simulink model "LQR"  (R2024b)
settings: Solver=VariableStepAuto  StartTime=0.0  StopTime=20  RelTol=1e-3
settings Model: Creator=12625  LastModifiedBy=12625

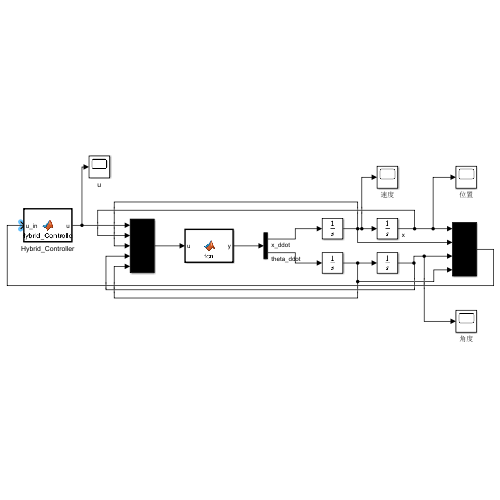
[thumbnail: Simulink's stored preview of the top-level diagram]
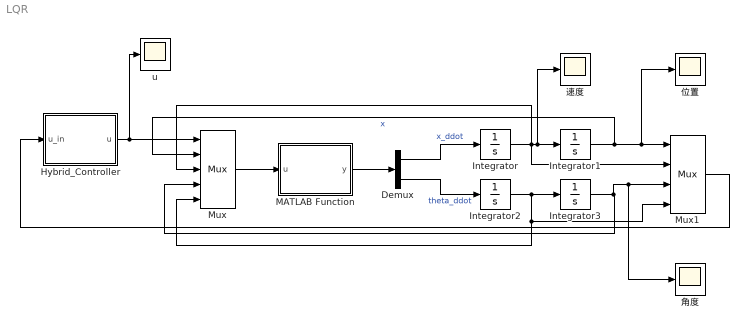
== system LQR ==
  Demux : Demux  Outputs=2
  Hybrid_Controller : MATLAB Function  TreatAsAtomicUnit=on
  Integrator : Integrator
  Integrator1 : Integrator
  Integrator2 : Integrator
  Integrator3 : Integrator  InitialCondition=-3.14
  MATLAB Function : MATLAB Function  TreatAsAtomicUnit=on
  Mux : Mux  Inputs=5
  Mux1 : Mux
  u : Scope
  位置 : Scope
  角度 : Scope
  速度 : Scope
  wires:
  Demux/1 -> Integrator/1  "x_ddot"
  Integrator/1 -> Mux1/2, Mux/3, 速度/1, Integrator1/1
  Demux/2 -> Integrator2/1  "theta_ddot"
  Integrator2/1 -> Mux1/4, Mux/5, Integrator3/1
  MATLAB Function/1(y) -> Demux/1
  Integrator1/1 -> 位置/1, Mux1/1, Mux/2  "x"
  Integrator3/1 -> 角度/1, Mux1/3, Mux/4
  Mux1/1 -> Hybrid_Controller/1(u_in)
  Hybrid_Controller/1(u) -> u/1, Mux/1
  Mux/1 -> MATLAB Function/1(u)

== matlab function LQR/MATLAB Function ==
  data: y output; u input
function y = fcn(u)
% 输入 u 包含: [F, x, x_dot, theta, theta_dot]
% 输出 y 包含: [x_ddot, theta_ddot]

% 1. 解包输入
F = u(1);
% x = u(2); % 其实方程里没用到x，只需要速度和角度
x_dot = u(3);
theta = u(4);
theta_dot = u(5);

% 2. 定义参数 (一定要和你的推导一致)
M = 1.0;  % 小车质量
m = 0.1;  % 摆杆质量
l = 0.5;  % 杆长的一半
g = 9.8;
I = 0.005; % 假设均匀杆 I = 1/12*m*(2l)^2 approx

% 3. 写入刚才推导出的公式 (这里用标准形式)
% 这里的公式是为了解出 x_ddot 和 theta_ddot
% 我们可以构建一个矩阵方程 Ax=b 来解，或者直接写解析解
% 为了简单，这里直接写解好的形式 (分母项)

sin_t = sin(theta);
cos_t = cos(theta);
denom = (M+m)*(I+m*l^2) - (m*l*cos_t)^2;

% 分子项
term1 = (I+m*l^2)*F + (I+m*l^2)*m*l*theta_dot^2*sin_t - m*l*cos_t*m*g*sin_t;
term2 = (M+m)*m*g*sin_t - m*l*cos_t*F - m*l*cos_t*m*l*theta_dot^2*sin_t;

x_ddot = term1 / denom;
theta_ddot = term2 / denom;

y = [x_ddot; theta_ddot];

== matlab function LQR/Hybrid_Controller ==
  data: u output; u_in input
function u = Hybrid_Controller(u_in)
    % 解包输入
    x = u_in(1);
    x_dot = u_in(2);
    theta = u_in(3);     % 原始角度
    theta_dot = u_in(4);
    
    % --- 1. 参数定义 ---
    M = 1.0; m = 0.1; l = 0.5; g = 9.8;
    I_cm = 0.005;
    J = I_cm + m*l^2;
    
    % --- 2. 角度归一化 ---
    theta_norm = mod(theta + pi, 2*pi) - pi;
    
    % --- 3. 能量计算 ---
    E_ref = m * g * l; 
    E_now = 0.5 * J * theta_dot^2 + m * g * l * cos(theta_norm);
    E_err = E_now - E_ref;

    clamp_val = 0.2; 
    E_err_safe = max(min(E_err, clamp_val), -clamp_val);
    
    % --- 4. 状态机切换逻辑 ---
    if abs(theta_norm) < 0.45
        % === 状态 A: LQR 稳态控制 ===
        K = [-1.0000   ,-3.4655  ,-73.5731  ,-11.5865]; 
        
        state_vec = [x; x_dot; theta_norm; theta_dot];
        u = -K * state_vec;
        
        % LQR 限幅
        u = max(min(u, 20), -20);
        
    else
        % === 状态 B: Swing-Up 起摆控制 (能量注入法) ===
        
        % 1. 计算能量注入项 (关键修改)
        % 原理：为了增加能量，力 F 的方向必须与 (theta_dot * cos(theta)) 一致
        % 这里的 E_err 通常是负数 (当前能量 < 目标能量)
        % 调节 k_swing 的大小决定起摆快慢
        k_swing = 300.0;  % 如果摆动太慢，把这个改大，比如 20 或 30
        
        % 使用平滑的控制律，而不是 sign()
        u_swing = k_swing * E_err * theta_dot * cos(theta_norm);
        
        % 2. 这里的符号非常关键！(试错点)
        u = u_swing; 
        
        % 3. 给小车位置加一个“软约束” (解决小车漂移问题)
        % 起摆时，小车很容易跑偏。加一点点 x 和 x_dot 的反馈把它拉住
        % 这里的系数不要太大，否则会干扰起摆
        k_pos = 1.0;
        k_vel = 0.5;
        u = u - (k_pos * x + k_vel * x_dot);

        % 4. 限幅
        u = max(min(u, 30), -30); %稍微给大一点力，25可能不够
    end
end
